simulink model "ParentApp"  (R2023a)
settings: Solver=FixedStepAuto  StartTime=0.0  StopTime=inf  RelTol=1e-3
undefined symbols (not defined in the file or in its folder): Audio_File_Write, TCP_IP
libraries: androidaudiovideolib x6, androidcommunicationlib x6, androiduilib x2, visionsources x1
settings Model: Creator=Nihar  LastModifiedBy=Hitesh
settings OptimizationCC: EnhancedBackFolding=on  PassReuseOutputArgsAs=Individual arguments  ZeroExternalMemoryAtStartup=off  ZeroInternalMemoryAtStartup=off  MaxStackSize=64  OptimizeBlockOrder=speed  DifferentSizesBufferReuse=on  OptimizationCustomize=off  EfficientTunableParamExpr=on
settings DebuggingCC: ParameterTunabilityLossMsg=error
settings HardwareCC: ProdBitPerLong=64  ProdLargestAtomicInteger=LongLong  ProdLargestAtomicFloat=Double  ProdLongLongMode=on  ProdHWDeviceType=ARM Compatible->ARM 64-bit (LP64)  UseEmbeddedCoderFeatures=off  UseSimulinkCoderFeatures=off
settings SFSimCC: MATLABDynamicMemAlloc=off
settings RTWCC: Description=Embedded Coder  SystemTargetFile=ert.tlc  HardwareBoard=Android Device (64bit)  TLCOptions="-aInlineSetEventsForThisBaseRateFcn=TLC_FALSE -aSuppressMultiTaskScheduler=TLC_FALSE  -aRateBasedStepFcn=0"  TemplateMakefile=ert_default_tmf  RTWVerbose=off  Toolchain=Android SDK/NDK Tools
settings CodeAppCC: ForceParamTrailComments=on  IgnoreCustomStorageClasses=off  OperatorAnnotations=on  SimulinkDataObjDesc=on  SFDataObjDesc=on  InsertBlockDesc=on
settings ERTTargetCC: SupportNonInlinedSFcns=on

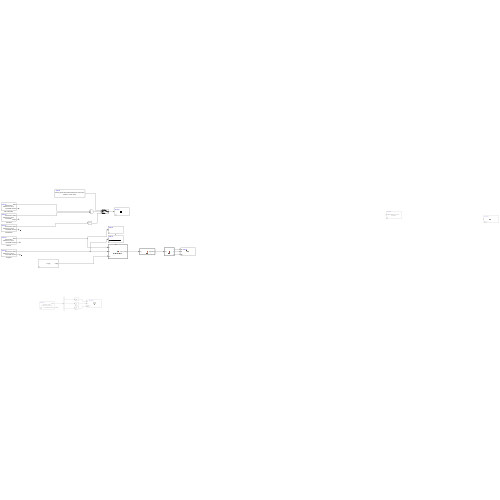
[thumbnail: Simulink's stored preview of the top-level diagram]
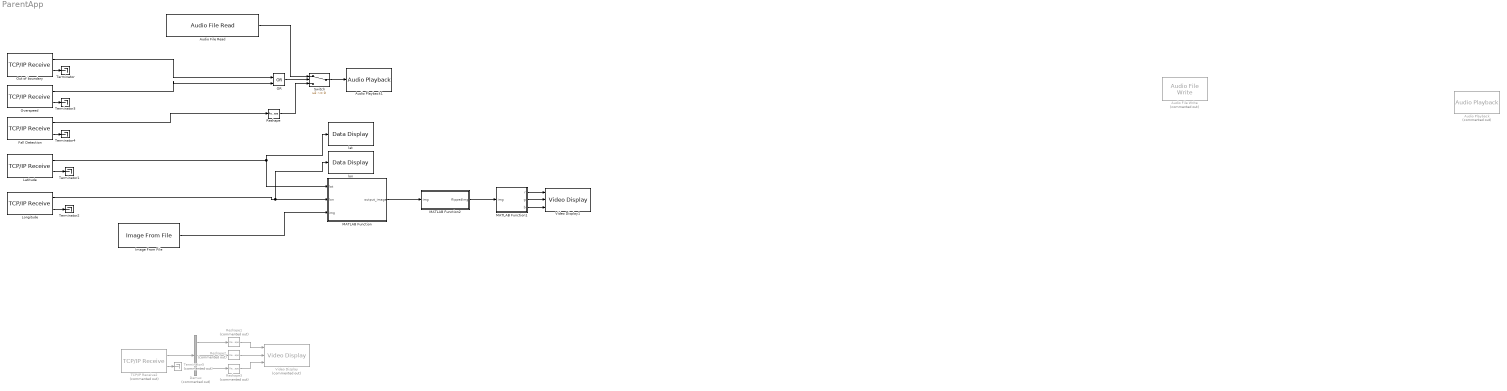
== system ParentApp ==
  Audio File Read : androidaudiovideolib/Audio File Read  FileName=C:\Users\Hitesh\Downloads\warning-buzzer-alarm-fascinatedsound-1-00-18.mp3  FrameSize=4410
  Audio File Write : androidaudiovideolib/Audio File Write  Commented=on  FileName=recordedsound  FileType=wav  AudioSamplingFreq=44100  RecordTimeControl=Block dialog  MaxRecordTime=60  BitRate=128  AudioFileWriteId=TCP_IP/Audio_File_Write
  Audio Playback : androidaudiovideolib/Audio Playback  Commented=on  SampleFreq=24000  AudioSamplingFreq=24000  SampleTime=0.1  DeviceStr=0  QueueDuration=0  BlockPlatform=Android
  Audio Playback1 : androidaudiovideolib/Audio Playback  SampleFreq=44100  AudioSamplingFreq=44100  SampleTime=0.1  DeviceStr=0  QueueDuration=0  BlockPlatform=Android
  Demux : Demux  Commented=on  Outputs=3
  Fall Detection : androidcommunicationlib/TCP//IP Receive  TCPReceiveId=ParentApp/Fall_Detection  Mode_=Client  LocalServerPort_=25000  RemoteAddr_=10.7.14.91  RemoteServerPort_=20000  DataType_=int16  DataSize_=8820  SampleTime_=0.1  ClientPortBindingSelection_=off  ClientPortToBind_=35000  BlockingMode_=off  BlockTimeout_=0.1
  Image From File : visionsources/Image From File  Tag=vipblks_nd  FileName=C:\Users\Hitesh\Downloads\TL.png  Ts=inf  imagePorts=One multidimensional signal  OutPortLabels=R|G|B  ImageDataType=uint8  sdImageDataType=uint(8)  Signed=on  WordLength=16  FractionLengthMode=User-defined  FractionLength=15
  Latitude : androidcommunicationlib/TCP//IP Receive  TCPReceiveId=ParentApp/Overspeed1  Mode_=Client  LocalServerPort_=25000  RemoteAddr_=10.7.14.91  RemoteServerPort_=50000  DataType_=double  DataSize_=1  SampleTime_=0.1  ClientPortBindingSelection_=off  ClientPortToBind_=35000  BlockingMode_=off  BlockTimeout_=0.1
  Longitude : androidcommunicationlib/TCP//IP Receive  TCPReceiveId=ParentApp/Overspeed2  Mode_=Client  LocalServerPort_=25000  RemoteAddr_=10.7.14.91  RemoteServerPort_=15000  DataType_=double  DataSize_=1  SampleTime_=0.1  ClientPortBindingSelection_=off  ClientPortToBind_=35000  BlockingMode_=off  BlockTimeout_=0.1
  MATLAB Function : MATLAB Function  TreatAsAtomicUnit=on
  MATLAB Function1 : MATLAB Function  TreatAsAtomicUnit=on
  MATLAB Function2 : MATLAB Function  TreatAsAtomicUnit=on
  OR : Logic  Operator=OR  IconShape=distinctive  AllPortsSameDT=off  OutDataTypeStr=boolean
  Out of boundary : androidcommunicationlib/TCP//IP Receive  TCPReceiveId=ParentApp/Out_of_boundary  Mode_=Client  LocalServerPort_=25000  RemoteAddr_=10.7.14.91  RemoteServerPort_=25000  DataType_=int16  DataSize_=1  SampleTime_=0.1  ClientPortBindingSelection_=off  ClientPortToBind_=35000  BlockingMode_=off  BlockTimeout_=0.1
  Overspeed : androidcommunicationlib/TCP//IP Receive  TCPReceiveId=ParentApp/Overspeed  Mode_=Client  LocalServerPort_=25000  RemoteAddr_=10.7.14.91  RemoteServerPort_=25500  DataType_=int16  DataSize_=1  SampleTime_=0.1  ClientPortBindingSelection_=off  ClientPortToBind_=35000  BlockingMode_=off  BlockTimeout_=0.1
  Reshape : Reshape  OutputDimensionality=Customize  OutputDimensions=[4410,2]
  Reshape1 : Reshape  Commented=on  OutputDimensionality=Customize  OutputDimensions=[320,240]
  Reshape2 : Reshape  Commented=on  OutputDimensionality=Customize  OutputDimensions=[320,240]
  Reshape3 : Reshape  Commented=on  OutputDimensionality=Customize  OutputDimensions=[320,240]
  Switch : Switch  Criteria=u2 ~= 0  SaturateOnIntegerOverflow=off  InputSameDT=off
  TCP/IP Receive2 : androidcommunicationlib/TCP//IP Receive  Commented=on  TCPReceiveId=ParentApp/TCP//IP_Receive2  Mode_=Client  LocalServerPort_=25000  RemoteAddr_=10.7.14.91  RemoteServerPort_=45000  DataType_=uint8  DataSize_=307200*3  SampleTime_=2  ClientPortBindingSelection_=off  ClientPortToBind_=35000  BlockingMode_=off  BlockTimeout_=0.1
  Terminator{,1..4} (5 alike) : Terminator
  Terminator5 : Terminator  Commented=on
  Video Display : androidaudiovideolib/Video Display  Commented=on  BlockPlatform=Android
  Video Display1 : androidaudiovideolib/Video Display  BlockPlatform=Android
  lat : androiduilib/Data Display  DataDisplayId=ParentApp/lat  Format=Float  Precision=6  SimulateUsing=Code generation  blockPlatform=Android
  lon : androiduilib/Data Display  DataDisplayId=ParentApp/lon  Format=Float  Precision=6  SimulateUsing=Code generation  blockPlatform=Android
  wires:
  TCP/IP Receive2/1 -> Demux/1
  Out of boundary/1 -> OR/1
  Overspeed/1 -> OR/2
  Fall Detection/1 -> Reshape/1
  Out of boundary/2 -> Terminator/1
  Audio File Read/1 -> Switch/1
  Reshape2/1 -> Video Display/2
  Reshape/1 -> Switch/3
  Reshape3/1 -> Video Display/3
  OR/1 -> Switch/2
  Demux/1 -> Reshape1/1
  Demux/2 -> Reshape2/1
  Demux/3 -> Reshape3/1
  Switch/1 -> Audio Playback1/1
  Reshape1/1 -> Video Display/1
  Longitude/1 -> lon/1, MATLAB Function/2(lon)
  Latitude/1 -> lat/1, MATLAB Function/1(lat)
  MATLAB Function/1(output_image) -> MATLAB Function2/1(img)
  MATLAB Function1/2(g) -> Video Display1/2
  MATLAB Function1/1(r) -> Video Display1/1
  MATLAB Function1/3(b) -> Video Display1/3
  Image From File/1 -> MATLAB Function/3(img)
  Latitude/2 -> Terminator1/1
  Longitude/2 -> Terminator2/1
  Overspeed/2 -> Terminator3/1
  Fall Detection/2 -> Terminator4/1
  MATLAB Function2/1(flippedImg) -> MATLAB Function1/1(img)
  TCP/IP Receive2/2 -> Terminator5/1

== matlab function ParentApp/MATLAB Function1 ==
  data: img input; r output; g output; b output
function [r,g,b] = fcn(img)
    r = img(:,:,1);
    g = img(:,:,2);
    b = img(:,:,3);
end

== matlab function ParentApp/MATLAB Function ==
  data: lat input; lon input; output_image output; img input
function output_image  = image_mapping(lat,lon,img)
    map_width = 883;
    map_height = 675;
    X = [83, 620, 640, 80, 441];
    Lx = [23.211144, 23.211170, 23.209616, 23.209530, 23.209997];
    Y = [70, 61, 427, 444, 337];
    Ly = [72.6833273, 72.685835, 72.685929, 72.683318, 72.685008];
    
    yL = zeros(map_height, 1);
    xL = zeros(1,map_width);

    for y = 1:map_height
            w_Y = ((y - Y(2)) * (y - Y(3)) * (y - Y(4)) * (y - Y(5))) / ((Y(1) - Y(2)) * (Y(1) - Y(3)) * (Y(1) - Y(4)) * (Y(1) - Y(5)));
            w_Y1 = ((y - Y(1)) * (y - Y(3)) * (y - Y(4)) * (y - Y(5))) / ((Y(2) - Y(1)) * (Y(2) - Y(3)) * (Y(2) - Y(4)) * (Y(2) - Y(5)));
            w_Y2 = ((y - Y(1)) * (y - Y(2)) * (y - Y(4)) * (y - Y(5))) / ((Y(3) - Y(1)) * (Y(3) - Y(2)) * (Y(3) - Y(4)) * (Y(3) - Y(5)));
            w_Y3 = ((y - Y(1)) * (y - Y(2)) * (y - Y(3)) * (y - Y(5))) / ((Y(4) - Y(1)) * (Y(4) - Y(2)) * (Y(4) - Y(3)) * (Y(4) - Y(5)));
            w_Y4 = ((y - Y(1)) * (y - Y(2)) * (y - Y(3)) * (y - Y(4))) / ((Y(5) - Y(1)) * (Y(5) - Y(2)) * (Y(5) - Y(3)) * (Y(5) - Y(4)));
            yL(y) = (w_Y * Lx(1)) + (w_Y1 * Lx(2)) + (w_Y2 * Lx(3)) + (w_Y3 * Lx(4)) + (w_Y4 * Lx(5));

    end
    for x = 1:map_width
            w_X = ((x - X(2)) * (x - X(3)) * (x - X(4)) * (x - X(5))) / ((X(1) - X(2)) * (X(1) - X(3)) * (X(1) - X(4)) * (X(1) - X(5)));
            w_X1 = ((x - X(1)) * (x - X(3)) * (x - X(4)) * (x - X(5))) / ((X(2) - X(1)) * (X(2) - X(3)) * (X(2) - X(4)) * (X(2) - X(5)));
            w_X2 = ((x - X(1)) * (x - X(2)) * (x - X(4)) * (x - X(5))) / ((X(3) - X(1)) * (X(3) - X(2)) * (X(3) - X(4)) * (X(3) - X(5)));
            w_X3 = ((x - X(1)) * (x - X(2)) * (x - X(3)) * (x - X(5))) / ((X(4) - X(1)) * (X(4) - X(2)) * (X(4) - X(3)) * (X(4) - X(5)));
            w_X4 = ((x - X(1)) * (x - X(2)) * (x - X(3)) * (x - X(4))) / ((X(5) - X(1)) * (X(5) - X(2)) * (X(5) - X(3)) * (X(5) - X(4)));
            xL(x) = (w_X * Ly(1)) + (w_X1 * Ly(2)) + (w_X2 * Ly(3)) + (w_X3 * Ly(4)) + (w_X4 * Ly(5));
     end
    
   
    
   
    [~, idx_y] = min(abs(yL - lat));
    [~, idx_x] = min(abs(xL - lon));
    min(abs(xL-lon))
    Xi = idx_x;
   
    Yi = idx_y;
    
    output_image = img;
    circle_radius = 7;
    % Ensure the circle coordinates are within bounds
    
    x = max(min(round(Xi), map_width), 1);
    y = max(min(round(Yi), map_height), 1);
    

    % Draw the filled circle manually
    for i = max(1, y - circle_radius):min(map_height, y + circle_radius)
        for j = max(1, x - circle_radius):min(map_width, x + circle_radius)
            if ((i - y)^2 + (j - x)^2) <= circle_radius^2
                output_image(i, j, 1) = 0; % Red channel
                output_image(i, j, 2) = 233;   % Green channel
                output_image(i, j, 3) = 226;   % Blue channel
            end
        end
    end
end

== matlab function ParentApp/MATLAB Function2 ==
  data: img input; flippedImg output
function flippedImg = flip(img)
    flippedImg = img(:, end:-1:1, :);
end
